simulink model "ICE_sim"  (R2026a)
settings: Solver=VariableStepAuto
PreLoadFcn:
  | % 模型加载前优先将当前目录与父目录加入 MATLAB 路径
  | modelPath = get_param(bdroot, 'FileName');
  | if ~isempty(modelPath)
  |     modelDir = fileparts(modelPath);
  |     addpath(modelDir);
  |     addpath(fullfile(modelDir, '..'));
  | end
InitFcn:
  | % 仅保留参数加载
  | common_params_init;
  | ice_params_init;
values from neighbouring files (symbols this model uses):
  BSFC_kg_per_kWh = Simulink.Parameter(0.24)    [ice_params_init.m]
  Critical_Overheat_Threshold_C = Simulink.Parameter(135)    [ice_params_init.m]
  Driveline_Efficiency = Simulink.Parameter(0.95)    [ice_params_init.m]
  Engine_HeatLossCoeff = Simulink.Parameter(0.1)    [ice_params_init.m]
  Engine_Temp_Init_C = Simulink.Parameter(40)    [ice_params_init.m]
  Engine_ThermalMass_JperC = Simulink.Parameter(50000)    [ice_params_init.m]
  Final_Drive_Ratio = Simulink.Parameter(3.5)    [ice_params_init.m]
  Fuel_Cut_RPM_Threshold = Simulink.Parameter(5000)    [ice_params_init.m]
  Fuel_Cut_Throttle_Threshold = Simulink.Parameter(5)    [ice_params_init.m]
  Fuel_Flow_Max_kg_s = Simulink.Parameter(0.028)    [ice_params_init.m]
  Fuel_LHV_J_per_kg = Simulink.Parameter(44e6)    [ice_params_init.m]
  Gear_Ratios = Simulink.Parameter([2.9 2.4 2.0 1.7 1.45 1.25 1.1 1.0])    [ice_params_init.m]
  Heat_Fraction_Coeff = Simulink.Parameter(0.3)    [ice_params_init.m]
  ICE_Max_Power_W = Simulink.Parameter(400000)    [ice_params_init.m]
  ICE_Max_Torque_Nm = Simulink.Parameter(320)    [ice_params_init.m]
  Idle_RPM_Threshold = Simulink.Parameter(4000)    [ice_params_init.m]
  Max_Safe_Boost_kPa = Simulink.Parameter(250)    [ice_params_init.m]
  Overheat_Threshold_C = Simulink.Parameter(105)    [ice_params_init.m]
  Race_Fuel_Limit_kg = Simulink.Parameter(110)    [ice_params_init.m]
  Shift_Down_RPM = Simulink.Parameter(9000)    [ice_params_init.m]
  Shift_Up_RPM = Simulink.Parameter(14500)    [ice_params_init.m]
  Throttle_Actuator_TimeConstant_s = Simulink.Parameter(0.05)    [ice_params_init.m]
  Turbo_FeedForward_Gain_Kff = Simulink.Parameter(1.0)    [ice_params_init.m]
  Turbo_FeedForward_Gain_Kff_Boosted = Simulink.Parameter(1.2)    [ice_params_init.m]
  Turbo_PID_Ki = Simulink.Parameter(0.1)    [ice_params_init.m]
  Turbo_PID_Kp = Simulink.Parameter(0.5)    [ice_params_init.m]
undefined symbols (not defined in the file or in its folder): Ambient_Temp_C, Wheel_Radius_m
libraries: simulink x1, sl_discontinuities x1, slpidlib x1
settings Model: Creator=nixiaofeng  LastModifiedBy=nixiaofeng

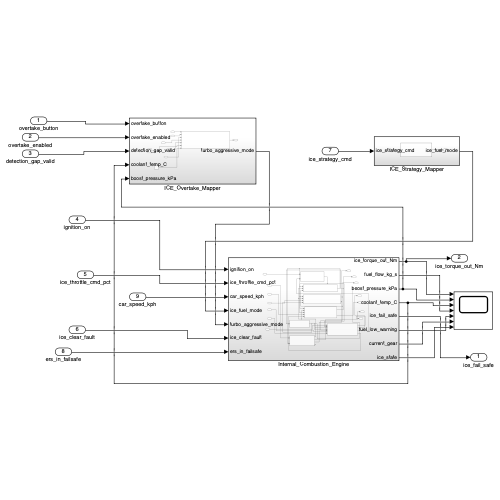
[thumbnail: Simulink's stored preview of the top-level diagram]
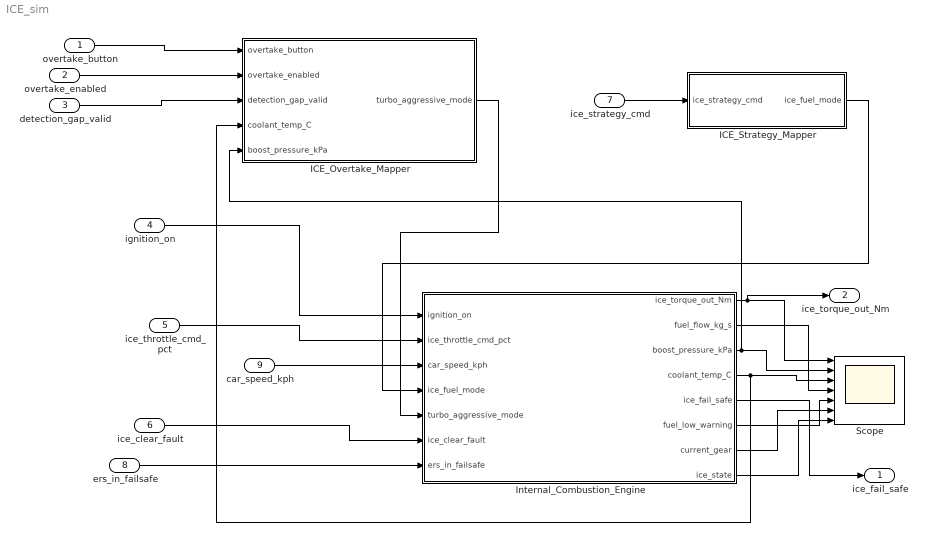
== system ICE_sim ==
  overtake_button : Inport
  overtake_enabled : Inport  Port=2
  detection_gap_valid : Inport  Port=3
  ignition_on : Inport  Port=4
  ice_throttle_cmd_pct : Inport  Port=5
  ice_clear_fault : Inport  Port=6
  ice_strategy_cmd : Inport  Port=7
  ers_in_failsafe : Inport  Port=8
  car_speed_kph : Inport  Port=9
  ICE_Overtake_Mapper : Subsystem
  ICE_Strategy_Mapper : Subsystem
  Internal_Combustion_Engine : Subsystem
  Scope : Scope  NumInputPorts=7
      settings: ActiveDisplayYMinimum=-5.6320436426453142  ActiveDisplayYMaximum=16.057146643170498
  ice_fail_safe : Outport
  ice_torque_out_Nm : Outport  Port=2
  wires:
  Internal_Combustion_Engine/1(ice_torque_out_Nm) -> ice_torque_out_Nm/1, Scope/1
  Internal_Combustion_Engine/3(boost_pressure_kPa) -> Scope/2, ICE_Overtake_Mapper/5(boost_pressure_kPa)
  Internal_Combustion_Engine/4(coolant_temp_C) -> ICE_Overtake_Mapper/4(coolant_temp_C), Scope/3
  Internal_Combustion_Engine/6(fuel_low_warning) -> Scope/5
  Internal_Combustion_Engine/2(fuel_flow_kg_s) -> Scope/4
  Internal_Combustion_Engine/7(current_gear) -> Scope/6
  Internal_Combustion_Engine/8(ice_state) -> Scope/7
  ICE_Strategy_Mapper/1(ice_fuel_mode) -> Internal_Combustion_Engine/4(ice_fuel_mode)
  ICE_Overtake_Mapper/1(turbo_aggressive_mode) -> Internal_Combustion_Engine/5(turbo_aggressive_mode)
  Internal_Combustion_Engine/5(ice_fail_safe) -> ice_fail_safe/1
  overtake_button/1 -> ICE_Overtake_Mapper/1(overtake_button)
  overtake_enabled/1 -> ICE_Overtake_Mapper/2(overtake_enabled)
  detection_gap_valid/1 -> ICE_Overtake_Mapper/3(detection_gap_valid)
  ignition_on/1 -> Internal_Combustion_Engine/1(ignition_on)
  ice_throttle_cmd_pct/1 -> Internal_Combustion_Engine/2(ice_throttle_cmd_pct)
  ice_clear_fault/1 -> Internal_Combustion_Engine/6(ice_clear_fault)
  ice_strategy_cmd/1 -> ICE_Strategy_Mapper/1(ice_strategy_cmd)
  ers_in_failsafe/1 -> Internal_Combustion_Engine/7(ers_in_failsafe)
  car_speed_kph/1 -> Internal_Combustion_Engine/3(car_speed_kph)

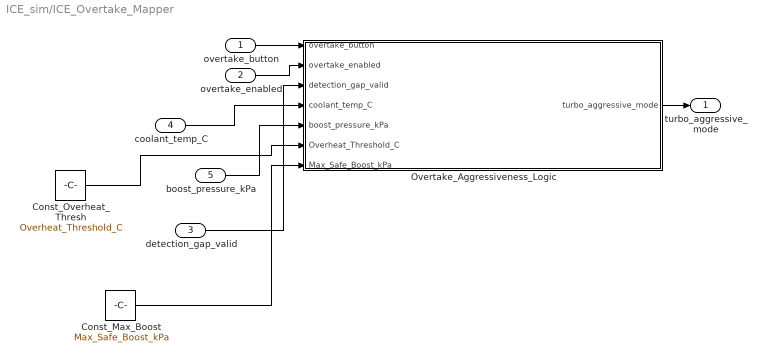
== system ICE_sim/ICE_Overtake_Mapper ==
  overtake_button : Inport
  overtake_enabled : Inport  Port=2
  detection_gap_valid : Inport  Port=3
  coolant_temp_C : Inport  Port=4
  boost_pressure_kPa : Inport  Port=5
  Const_Max_Boost : Constant  Value=Max_Safe_Boost_kPa
  Const_Overheat_Thresh : Constant  Value=Overheat_Threshold_C
  Overtake_Aggressiveness_Logic : MATLAB Function  TreatAsAtomicUnit=on
  turbo_aggressive_mode : Outport
  wires:
  overtake_button/1 -> Overtake_Aggressiveness_Logic/1(overtake_button)
  overtake_enabled/1 -> Overtake_Aggressiveness_Logic/2(overtake_enabled)
  detection_gap_valid/1 -> Overtake_Aggressiveness_Logic/3(detection_gap_valid)
  coolant_temp_C/1 -> Overtake_Aggressiveness_Logic/4(coolant_temp_C)
  boost_pressure_kPa/1 -> Overtake_Aggressiveness_Logic/5(boost_pressure_kPa)
  Const_Overheat_Thresh/1 -> Overtake_Aggressiveness_Logic/6(Overheat_Threshold_C)
  Const_Max_Boost/1 -> Overtake_Aggressiveness_Logic/7(Max_Safe_Boost_kPa)
  Overtake_Aggressiveness_Logic/1(turbo_aggressive_mode) -> turbo_aggressive_mode/1

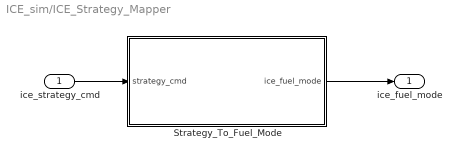
== system ICE_sim/ICE_Strategy_Mapper ==
  ice_strategy_cmd : Inport
  Strategy_To_Fuel_Mode : MATLAB Function  TreatAsAtomicUnit=on
  ice_fuel_mode : Outport
  wires:
  ice_strategy_cmd/1 -> Strategy_To_Fuel_Mode/1(strategy_cmd)
  Strategy_To_Fuel_Mode/1(ice_fuel_mode) -> ice_fuel_mode/1

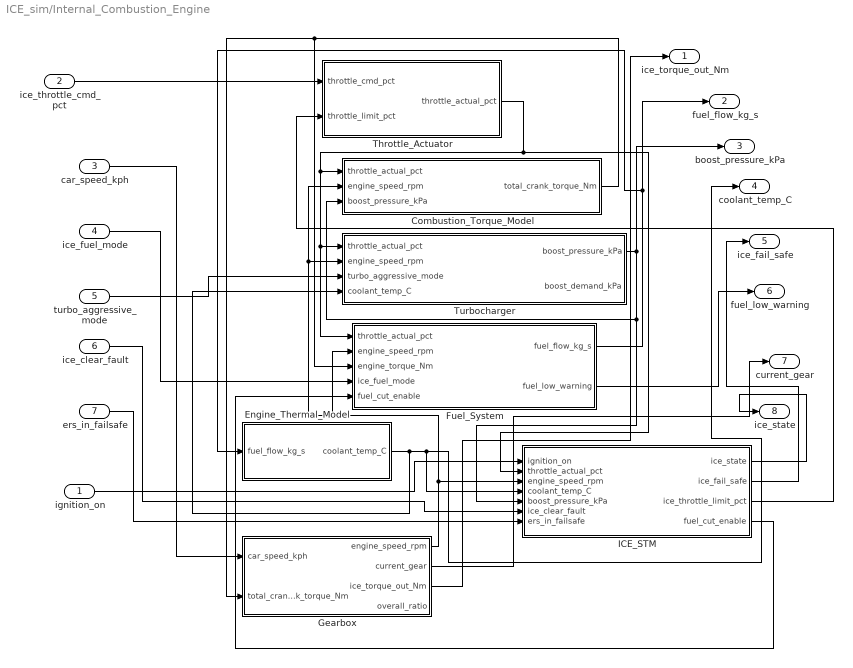
== system ICE_sim/Internal_Combustion_Engine ==
  ignition_on : Inport  OutDataTypeStr=boolean
  ice_throttle_cmd_pct : Inport  Port=2
  car_speed_kph : Inport  Port=3
  ice_fuel_mode : Inport  Port=4
  turbo_aggressive_mode : Inport  Port=5  OutDataTypeStr=boolean
  ice_clear_fault : Inport  Port=6  OutDataTypeStr=boolean
  ers_in_failsafe : Inport  Port=7  OutDataTypeStr=boolean
  Combustion_Torque_Model : Subsystem
  Engine_Thermal_Model : Subsystem
  Fuel_System : Subsystem
  Gearbox : Subsystem
  ICE_STM : Subsystem
  Throttle_Actuator : Subsystem
  Turbocharger : Subsystem
  ice_torque_out_Nm : Outport
  fuel_flow_kg_s : Outport  Port=2
  boost_pressure_kPa : Outport  Port=3
  coolant_temp_C : Outport  Port=4
  ice_fail_safe : Outport  Port=5
  fuel_low_warning : Outport  Port=6
  current_gear : Outport  Port=7
  ice_state : Outport  Port=8
  wires:
  ice_throttle_cmd_pct/1 -> Throttle_Actuator/1(throttle_cmd_pct)
  Throttle_Actuator/1(throttle_actual_pct) -> ICE_STM/2(throttle_actual_pct), Fuel_System/1(throttle_actual_pct), Turbocharger/1(throttle_actual_pct), Combustion_Torque_Model/1(throttle_actual_pct)
  ICE_STM/3(ice_throttle_limit_pct) -> Throttle_Actuator/2(throttle_limit_pct)
  Gearbox/1(engine_speed_rpm) -> ICE_STM/3(engine_speed_rpm), Fuel_System/2(engine_speed_rpm), Turbocharger/2(engine_speed_rpm), Combustion_Torque_Model/2(engine_speed_rpm)
  ignition_on/1 -> ICE_STM/1(ignition_on)
  Turbocharger/1(boost_pressure_kPa) -> ICE_STM/5(boost_pressure_kPa), Combustion_Torque_Model/3(boost_pressure_kPa), boost_pressure_kPa/1
  turbo_aggressive_mode/1 -> Turbocharger/3(turbo_aggressive_mode)
  Combustion_Torque_Model/1(total_crank_torque_Nm) -> Fuel_System/3(engine_torque_Nm), Gearbox/2(total_crank_torque_Nm)
  car_speed_kph/1 -> Gearbox/1(car_speed_kph)
  Gearbox/3(ice_torque_out_Nm) -> ice_torque_out_Nm/1
  Gearbox/2(current_gear) -> current_gear/1
  ice_fuel_mode/1 -> Fuel_System/4(ice_fuel_mode)
  ICE_STM/4(fuel_cut_enable) -> Fuel_System/5(fuel_cut_enable)
  Fuel_System/1(fuel_flow_kg_s) -> Engine_Thermal_Model/1(fuel_flow_kg_s), fuel_flow_kg_s/1
  Fuel_System/2(fuel_low_warning) -> fuel_low_warning/1
  Engine_Thermal_Model/1(coolant_temp_C) -> Turbocharger/4(coolant_temp_C), ICE_STM/4(coolant_temp_C), coolant_temp_C/1
  ice_clear_fault/1 -> ICE_STM/6(ice_clear_fault)
  ers_in_failsafe/1 -> ICE_STM/7(ers_in_failsafe)
  ICE_STM/1(ice_state) -> ice_state/1
  ICE_STM/2(ice_fail_safe) -> ice_fail_safe/1

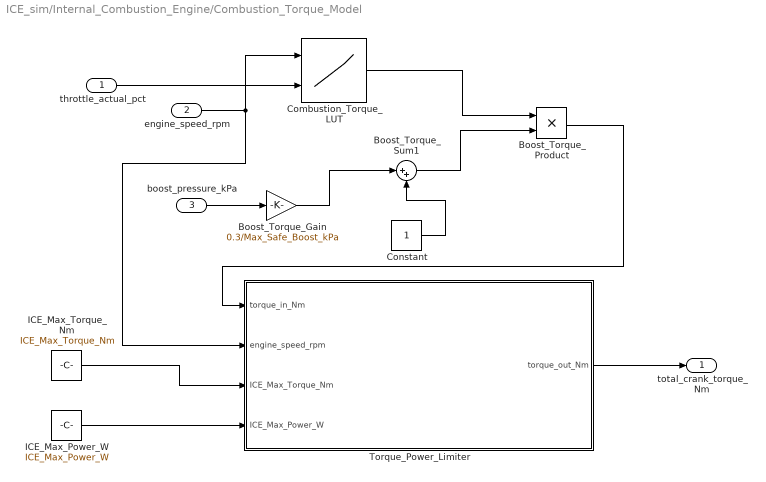
== system ICE_sim/Internal_Combustion_Engine/Combustion_Torque_Model ==
  throttle_actual_pct : Inport  Unit=%
  engine_speed_rpm : Inport  Port=2  Unit=rpm
  boost_pressure_kPa : Inport  Port=3  Unit=kPa
  Boost_Torque_Gain : Gain  Gain=0.3/Max_Safe_Boost_kPa
  Boost_Torque_Product : Product
  Boost_Torque_Sum1 : Sum  Inputs=|++
  Combustion_Torque_LUT : Lookup_n-D  BreakpointsForDimension1=[4000 6000 8000 10000 12000 14000 15000]  BreakpointsForDimension2=[0 20 40 60 80 100]  Table=|  InternalRulePriority=Speed  RndMeth=Simplest
      | [0 50 100 150 200 250;
      |  0 80 160 240 320 400;
      |  0 100 200 300 400 500;
      |  0 110 220 330 440 550;
      |  0 105 210 315 420 525;
      |  0 90 180 270 360 450;
      |  0 70 140 210 280 350]
      settings: InputPortMap=u0,u1
  Constant : Constant
  ICE_Max_Power_W : Constant  Value=ICE_Max_Power_W
  ICE_Max_Torque_Nm : Constant  Value=ICE_Max_Torque_Nm
  Torque_Power_Limiter : MATLAB Function  TreatAsAtomicUnit=on
  total_crank_torque_Nm : Outport  Unit=N*m
  wires:
  Constant/1 -> Boost_Torque_Sum1/2
  engine_speed_rpm/1 -> Torque_Power_Limiter/2(engine_speed_rpm), Combustion_Torque_LUT/1
  Combustion_Torque_LUT/1 -> Boost_Torque_Product/1
  boost_pressure_kPa/1 -> Boost_Torque_Gain/1
  Boost_Torque_Gain/1 -> Boost_Torque_Sum1/1
  Boost_Torque_Sum1/1 -> Boost_Torque_Product/2
  Torque_Power_Limiter/1(torque_out_Nm) -> total_crank_torque_Nm/1
  Boost_Torque_Product/1 -> Torque_Power_Limiter/1(torque_in_Nm)
  throttle_actual_pct/1 -> Combustion_Torque_LUT/2
  ICE_Max_Torque_Nm/1 -> Torque_Power_Limiter/3(ICE_Max_Torque_Nm)
  ICE_Max_Power_W/1 -> Torque_Power_Limiter/4(ICE_Max_Power_W)

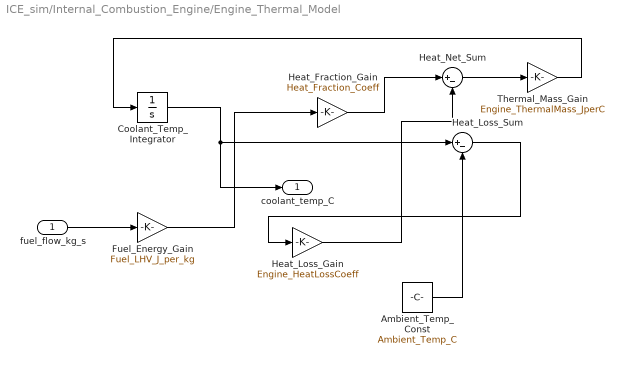
== system ICE_sim/Internal_Combustion_Engine/Engine_Thermal_Model ==
  fuel_flow_kg_s : Inport
  Ambient_Temp_Const : Constant  Value=Ambient_Temp_C
  Coolant_Temp_Integrator : Integrator  InitialCondition=Engine_Temp_Init_C
  Fuel_Energy_Gain : Gain  Gain=Fuel_LHV_J_per_kg
  Heat_Fraction_Gain : Gain  Gain=Heat_Fraction_Coeff
  Heat_Loss_Gain : Gain  Gain=Engine_HeatLossCoeff
  Heat_Loss_Sum : Sum  Inputs=|+-
  Heat_Net_Sum : Sum  Inputs=|+-
  Thermal_Mass_Gain : Gain  Gain=Engine_ThermalMass_JperC
  coolant_temp_C : Outport
  wires:
  fuel_flow_kg_s/1 -> Fuel_Energy_Gain/1
  Fuel_Energy_Gain/1 -> Heat_Fraction_Gain/1
  Heat_Fraction_Gain/1 -> Heat_Net_Sum/1
  Coolant_Temp_Integrator/1 -> coolant_temp_C/1, Heat_Loss_Sum/1
  Ambient_Temp_Const/1 -> Heat_Loss_Sum/2
  Heat_Loss_Sum/1 -> Heat_Loss_Gain/1
  Heat_Loss_Gain/1 -> Heat_Net_Sum/2
  Heat_Net_Sum/1 -> Thermal_Mass_Gain/1
  Thermal_Mass_Gain/1 -> Coolant_Temp_Integrator/1

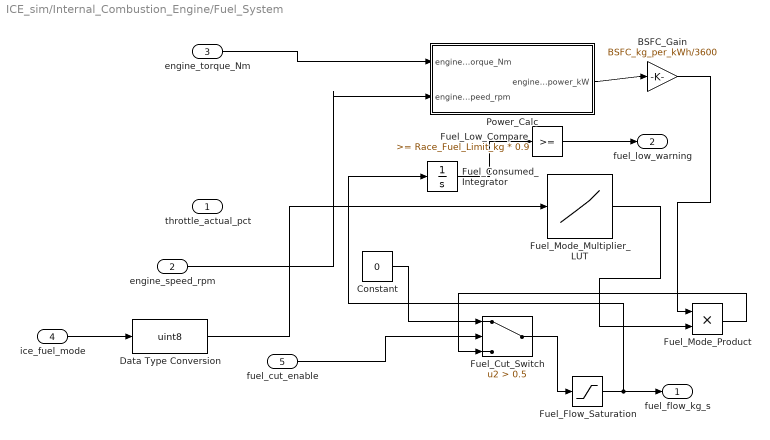
== system ICE_sim/Internal_Combustion_Engine/Fuel_System ==
  throttle_actual_pct : Inport
  engine_speed_rpm : Inport  Port=2
  engine_torque_Nm : Inport  Port=3
  ice_fuel_mode : Inport  Port=4
  fuel_cut_enable : Inport  Port=5
  BSFC_Gain : Gain  Gain=BSFC_kg_per_kWh/3600
  Constant : Constant  Value=0
  Data Type Conversion : DataTypeConversion  OutDataTypeStr=uint8  SaturateOnIntegerOverflow=off  RndMeth=Floor
  Fuel_Consumed_Integrator : Integrator
  Fuel_Cut_Switch : Switch  Criteria=u2 > Threshold  Threshold=0.5  SaturateOnIntegerOverflow=off  InputSameDT=off
  Fuel_Flow_Saturation : Saturate  UpperLimit=Fuel_Flow_Max_kg_s  LowerLimit=0
  Fuel_Low_Compare : simulink/Logic and Bit Operations/Compare To Constant  relop=>=  const=Race_Fuel_Limit_kg * 0.9  OutDataTypeStr=boolean
  Fuel_Mode_Multiplier_LUT : Lookup_n-D  NumberOfTableDimensions=1  BreakpointsForDimension1=[0 1 2]  BreakpointsForDimension1DataTypeStr=Inherit: Inherit from 'Breakpoint data'  Table=[1.0 0.75 0.55]  ExtrapMethod=Clip  InternalRulePriority=Speed  OutDataTypeStr=double  RndMeth=Simplest
  Fuel_Mode_Product : Product
  Power_Calc : Subsystem
  fuel_flow_kg_s : Outport
  fuel_low_warning : Outport  Port=2
  wires:
  engine_torque_Nm/1 -> Power_Calc/1(engine_torque_Nm)
  engine_speed_rpm/1 -> Power_Calc/2(engine_speed_rpm)
  Power_Calc/1(engine_power_kW) -> BSFC_Gain/1
  BSFC_Gain/1 -> Fuel_Mode_Product/1
  Fuel_Mode_Multiplier_LUT/1 -> Fuel_Mode_Product/2
  Constant/1 -> Fuel_Cut_Switch/1
  fuel_cut_enable/1 -> Fuel_Cut_Switch/2
  Fuel_Mode_Product/1 -> Fuel_Cut_Switch/3
  Fuel_Cut_Switch/1 -> Fuel_Flow_Saturation/1
  Fuel_Flow_Saturation/1 -> Fuel_Consumed_Integrator/1, fuel_flow_kg_s/1
  Fuel_Consumed_Integrator/1 -> Fuel_Low_Compare/1
  Fuel_Low_Compare/1 -> fuel_low_warning/1
  ice_fuel_mode/1 -> Data Type Conversion/1
  Data Type Conversion/1 -> Fuel_Mode_Multiplier_LUT/1

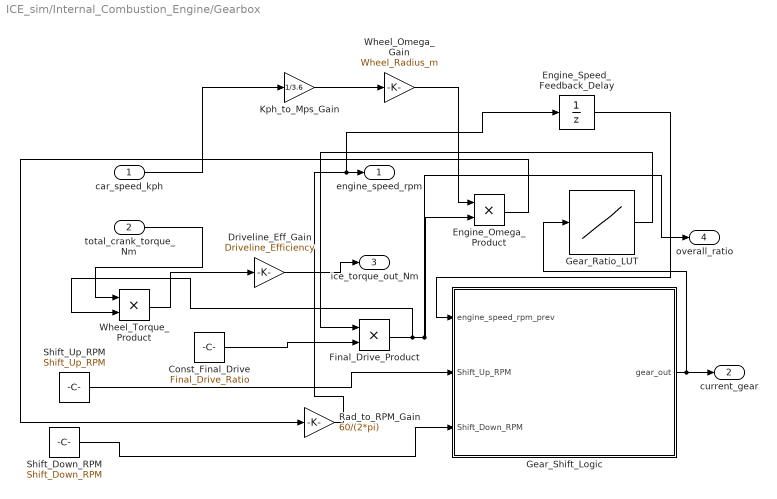
== system ICE_sim/Internal_Combustion_Engine/Gearbox ==
  car_speed_kph : Inport
  total_crank_torque_Nm : Inport  Port=2
  Const_Final_Drive : Constant  Value=Final_Drive_Ratio
  Driveline_Eff_Gain : Gain  Gain=Driveline_Efficiency
  Engine_Omega_Product : Product
  Engine_Speed_Feedback_Delay : UnitDelay  InitialCondition=Idle_RPM_Threshold  SampleTime=-1
  Final_Drive_Product : Product
  Gear_Ratio_LUT : Lookup_n-D  NumberOfTableDimensions=1  BreakpointsForDimension1=[1 2 3 4 5 6 7 8]  Table=Gear_Ratios  TableDataTypeStr=Inherit: Inherit from 'Table data'  ExtrapMethod=Clip  InternalRulePriority=Speed  OutDataTypeStr=double  RndMeth=Simplest
  Gear_Shift_Logic : MATLAB Function  TreatAsAtomicUnit=on
  Kph_to_Mps_Gain : Gain  Gain=1/3.6
  Rad_to_RPM_Gain : Gain  Gain=60/(2*pi)
  Shift_Down_RPM : Constant  Value=Shift_Down_RPM
  Shift_Up_RPM : Constant  Value=Shift_Up_RPM
  Wheel_Omega_Gain : Gain  Gain=Wheel_Radius_m
  Wheel_Torque_Product : Product
  engine_speed_rpm : Outport
  current_gear : Outport  Port=2
  ice_torque_out_Nm : Outport  Port=3
  overall_ratio : Outport  Port=4
  wires:
  Shift_Up_RPM/1 -> Gear_Shift_Logic/2(Shift_Up_RPM)
  Shift_Down_RPM/1 -> Gear_Shift_Logic/3(Shift_Down_RPM)
  Engine_Speed_Feedback_Delay/1 -> Gear_Shift_Logic/1(engine_speed_rpm_prev)
  Gear_Shift_Logic/1(gear_out) -> Gear_Ratio_LUT/1, current_gear/1
  Gear_Ratio_LUT/1 -> Final_Drive_Product/1
  Const_Final_Drive/1 -> Final_Drive_Product/2
  car_speed_kph/1 -> Kph_to_Mps_Gain/1
  Kph_to_Mps_Gain/1 -> Wheel_Omega_Gain/1
  Wheel_Omega_Gain/1 -> Engine_Omega_Product/1
  Final_Drive_Product/1 -> Wheel_Torque_Product/2, overall_ratio/1, Engine_Omega_Product/2
  Engine_Omega_Product/1 -> Rad_to_RPM_Gain/1
  Rad_to_RPM_Gain/1 -> Engine_Speed_Feedback_Delay/1, engine_speed_rpm/1
  total_crank_torque_Nm/1 -> Wheel_Torque_Product/1
  Wheel_Torque_Product/1 -> Driveline_Eff_Gain/1
  Driveline_Eff_Gain/1 -> ice_torque_out_Nm/1

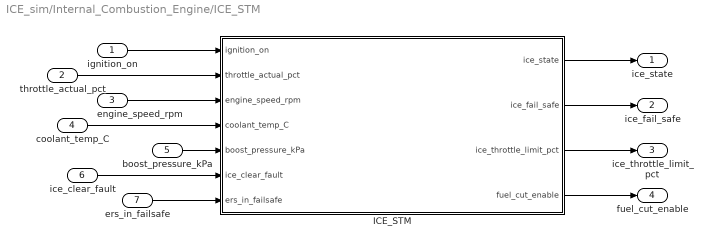
== system ICE_sim/Internal_Combustion_Engine/ICE_STM ==
  ignition_on : Inport
  throttle_actual_pct : Inport  Port=2
  engine_speed_rpm : Inport  Port=3
  coolant_temp_C : Inport  Port=4
  boost_pressure_kPa : Inport  Port=5
  ice_clear_fault : Inport  Port=6
  ers_in_failsafe : Inport  Port=7
  ICE_STM : Stateflow chart  TreatAsAtomicUnit=on
  ice_state : Outport
  ice_fail_safe : Outport  Port=2
  ice_throttle_limit_pct : Outport  Port=3
  fuel_cut_enable : Outport  Port=4
  wires:
  ignition_on/1 -> ICE_STM/1(ignition_on)
  throttle_actual_pct/1 -> ICE_STM/2(throttle_actual_pct)
  engine_speed_rpm/1 -> ICE_STM/3(engine_speed_rpm)
  coolant_temp_C/1 -> ICE_STM/4(coolant_temp_C)
  boost_pressure_kPa/1 -> ICE_STM/5(boost_pressure_kPa)
  ice_clear_fault/1 -> ICE_STM/6(ice_clear_fault)
  ers_in_failsafe/1 -> ICE_STM/7(ers_in_failsafe)
  ICE_STM/1(ice_state) -> ice_state/1
  ICE_STM/2(ice_fail_safe) -> ice_fail_safe/1
  ICE_STM/3(ice_throttle_limit_pct) -> ice_throttle_limit_pct/1
  ICE_STM/4(fuel_cut_enable) -> fuel_cut_enable/1

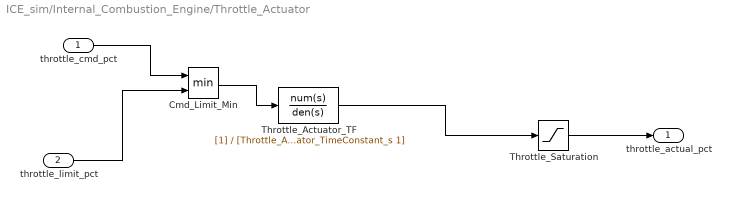
== system ICE_sim/Internal_Combustion_Engine/Throttle_Actuator ==
  throttle_cmd_pct : Inport  Unit=%
  throttle_limit_pct : Inport  Port=2  Unit=%
  Cmd_Limit_Min : MinMax  Inputs=2
  Throttle_Actuator_TF : TransferFcn  Denominator=[Throttle_Actuator_TimeConstant_s 1]
  Throttle_Saturation : Saturate  UpperLimit=100  LowerLimit=0
  throttle_actual_pct : Outport  Unit=%
  wires:
  throttle_cmd_pct/1 -> Cmd_Limit_Min/1
  throttle_limit_pct/1 -> Cmd_Limit_Min/2
  Cmd_Limit_Min/1 -> Throttle_Actuator_TF/1
  Throttle_Actuator_TF/1 -> Throttle_Saturation/1
  Throttle_Saturation/1 -> throttle_actual_pct/1

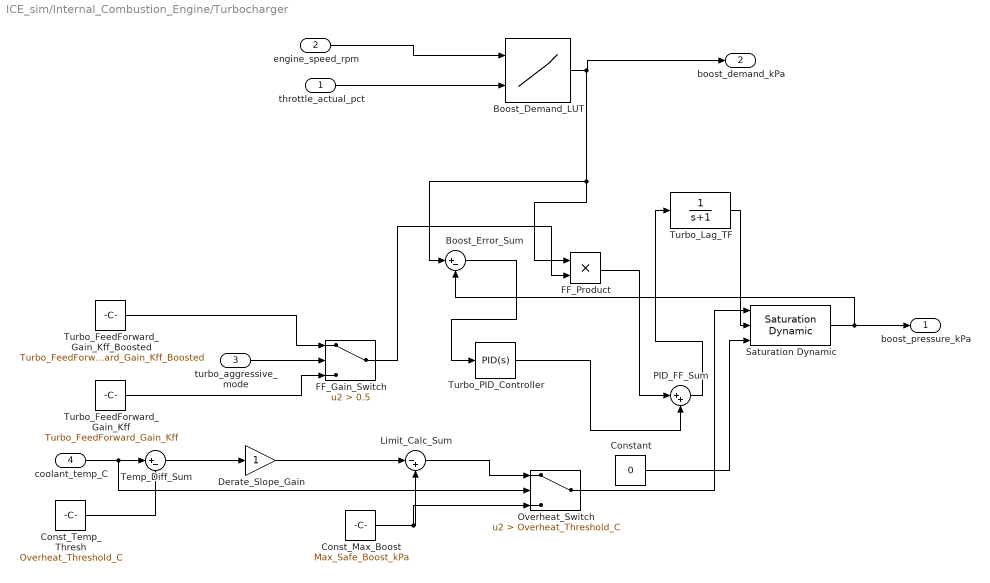
== system ICE_sim/Internal_Combustion_Engine/Turbocharger ==
  throttle_actual_pct : Inport
  engine_speed_rpm : Inport  Port=2
  turbo_aggressive_mode : Inport  Port=3
  coolant_temp_C : Inport  Port=4
  Boost_Demand_LUT : Lookup_n-D  BreakpointsForDimension1=[4000 6000 8000 10000 12000 14000 15000]  BreakpointsForDimension2=[0 20 40 60 80 100]  Table=|  InternalRulePriority=Speed  RndMeth=Simplest
      | [ 0  10   30   60   90  120;
      |   0  20   50  100  140  180;
      |   0  30   70  130  180  220;
      |   0  40   80  150  200  250;
      |   0  40   80  150  200  250;
      |   0  35   70  130  180  220;
      |   0  20   50  100  140  180 ]
      settings: InputPortMap=u0,u1
  Boost_Error_Sum : Sum  Inputs=|+-
  Const_Max_Boost : Constant  Value=Max_Safe_Boost_kPa
  Const_Temp_Thresh : Constant  Value=Overheat_Threshold_C
  Constant : Constant  Value=0
  Derate_Slope_Gain : Gain
  FF_Gain_Switch : Switch  Criteria=u2 > Threshold  Threshold=0.5  SaturateOnIntegerOverflow=off  InputSameDT=off
  FF_Product : Product
  Limit_Calc_Sum : Sum  Inputs=|-+
  Overheat_Switch : Switch  Criteria=u2 > Threshold  Threshold=Overheat_Threshold_C  SaturateOnIntegerOverflow=off  InputSameDT=off
  PID_FF_Sum : Sum  Inputs=|++
  Saturation Dynamic : sl_discontinuities/Saturation Dynamic  OutMin=[]  OutMax=[]  OutDataTypeStr=Inherit: Same as second input  OutDataType=fixdt(1, 16)  OutScaling=2^-10  DoSatur=off
      settings: LibrarySourceBlock=|
      | simulink/Discontinuities/Saturation
      | Dynamic
  Temp_Diff_Sum : Sum  Inputs=|+-
  Turbo_FeedForward_Gain_Kff : Constant  Value=Turbo_FeedForward_Gain_Kff
  Turbo_FeedForward_Gain_Kff_Boosted : Constant  Value=Turbo_FeedForward_Gain_Kff_Boosted
  Turbo_Lag_TF : TransferFcn  Denominator=[1 1]
  Turbo_PID_Controller : slpidlib/PID Controller  Controller=PID  Form=Parallel  TimeDomain=Continuous-time  UseExternalTs=off  SampleTime=-1  IntegratorMethod=Forward Euler  FilterMethod=Forward Euler  ControllerParametersSource=internal  P=Turbo_PID_Kp  I=Turbo_PID_Ki  UseKiTs=off  D=0  UseExternalDerivativeSource=off  N=100  UseFilter=on  TunerSelectOption=Transfer Function Based (PID Tuner App)  InitialConditionSource=internal  InitialConditionForIntegrator=0  InitialConditionForFilter=0  DifferentiatorICPrevScaledInput=0  ExternalReset=none  TrackingMode=off  Kt=1  LimitOutput=off  SatLimitsSource=internal  UpperSaturationLimit=inf  LowerSaturationLimit=-inf  LinearizeAsGain=on  AntiWindupMode=none  Kb=1  LimitIntegrator=off  UpperIntegratorSaturationLimit=inf  LowerIntegratorSaturationLimit=-inf  POutMin=[]  POutMax=[]  IOutMin=[]  IOutMax=[]  DOutMin=[]  DOutMax=[]  NOutMin=[]  NOutMax=[]  SumOutMin=[]  SumOutMax=[]  SaturationOutMin=[]  SaturationOutMax=[]  PParamMin=[]  PParamMax=[]  IParamMin=[]  IParamMax=[]  DParamMin=[]  DParamMax=[]  NParamMin=[]  NParamMax=[]  KbParamMin=[]  KbParamMax=[]  KtParamMin=[]  KtParamMax=[]  KbOutMin=[]  KbOutMax=[]  KtOutMin=[]  KtOutMax=[]  IntegratorOutMin=[]  IntegratorOutMax=[]  FilterOutMin=[]  FilterOutMax=[]  SumI1OutMin=[]  SumI1OutMax=[]  SumI2OutMin=[]  SumI2OutMax=[]  SumI3OutMin=[]  SumI3OutMax=[]  SumI4OutMin=[]  SumI4OutMax=[]  SumDOutMin=[]  SumDOutMax=[]  DifferentiatorOutMin=[]  DifferentiatorOutMax=[]  FilterDiffOutCoefMin=[]  FilterDiffOutCoefMax=[]  ReciprocalOutMin=[]  ReciprocalOutMax=[]  SumDenOutMin=[]  SumDenOutMax=[]  SumNumOutMin=[]  SumNumOutMax=[]  DivideOutMin=[]  DivideOutMax=[]  UdiffTsProdOutMin=[]  UdiffTsProdOutMax=[]  NTsProdOutMin=[]  NTsProdOutMax=[]  UintegralTsProdOutMin=[]  UintegralTsProdOutMax=[]  UngainTsProdOutMin=[]  UngainTsProdOutMax=[]  ClampingZeroOutDataTypeStr=Inherit: Inherit via back propagation  ClampingZeroOutMin=[]  ClampingZeroOutMax=[]  FilterDenConstantOutDataTypeStr=Inherit: Inherit via back propagation  FilterDenConstantOutMin=[]  FilterDenConstantOutMax=[]  PCopyOutDataTypeStr=Inherit: Inherit via back propagation  PCopyOutMin=[]  PCopyOutMax=[]  NCopyOutDataTypeStr=Inherit: Inherit via back propagation  NCopyOutMin=[]  NCopyOutMax=[]  IntegratorContinuousStateAttributes=''  IntegratorStateMustResolveToSignalObject=off  IntegratorRTWStateStorageClass=Auto  FilterContinuousStateAttributes=''  FilterStateMustResolveToSignalObject=off  FilterRTWStateStorageClass=Auto  ParallelPVariant=InternalParameters  IdealPVariant=Disabled  IVariant=InternalParameters  DVariant=InternalParameters  IntegratorVariant=Continuous  SatVariant=Disabled  AWVariant=Passthrough  PCopyVariant=Disabled  TRVariant=Disabled  FdbkBlocksVariant=Forward  IdealPFdbkVariant=Disabled  SatFdbkVariant=Disabled  DerivativeFilterVariant=ContFilter  NVariant=InternalParameters  NCopyVariant=Disabled  FilterICVariant=InternalICsFilter  IntegratorICVariant=InternalICs  ExternalResetVariant=Disabled  TRSumVariant=Passthrough  SumFdbkVariant=Disabled  SumVariant=Sum_PID  TsampFilterVariant=InternalTs  TsampNgainVariant=Passthrough  TsampIntegralVariant=Disabled_SignalSpec  ExternalSaturationOutDataTypeStr=Inherit: Same as second input  DerivativeSourceVariant=ErrorSignal  PreIntVariant=InternalPreInt
  boost_pressure_kPa : Outport
  boost_demand_kPa : Outport  Port=2
  wires:
  engine_speed_rpm/1 -> Boost_Demand_LUT/1
  throttle_actual_pct/1 -> Boost_Demand_LUT/2
  Boost_Demand_LUT/1 -> FF_Product/1, Boost_Error_Sum/1, boost_demand_kPa/1
  turbo_aggressive_mode/1 -> FF_Gain_Switch/2
  Turbo_FeedForward_Gain_Kff_Boosted/1 -> FF_Gain_Switch/1
  Turbo_FeedForward_Gain_Kff/1 -> FF_Gain_Switch/3
  Turbo_Lag_TF/1 -> Saturation Dynamic/2
  Saturation Dynamic/1 -> boost_pressure_kPa/1, Boost_Error_Sum/2
  Constant/1 -> Saturation Dynamic/3
  coolant_temp_C/1 -> Overheat_Switch/2, Temp_Diff_Sum/1
  Const_Temp_Thresh/1 -> Temp_Diff_Sum/2
  Temp_Diff_Sum/1 -> Derate_Slope_Gain/1
  Derate_Slope_Gain/1 -> Limit_Calc_Sum/1
  Const_Max_Boost/1 -> Overheat_Switch/3, Limit_Calc_Sum/2
  Limit_Calc_Sum/1 -> Overheat_Switch/1
  Overheat_Switch/1 -> Saturation Dynamic/1
  Boost_Error_Sum/1 -> Turbo_PID_Controller/1
  FF_Gain_Switch/1 -> FF_Product/2
  FF_Product/1 -> PID_FF_Sum/1
  Turbo_PID_Controller/1 -> PID_FF_Sum/2
  PID_FF_Sum/1 -> Turbo_Lag_TF/1

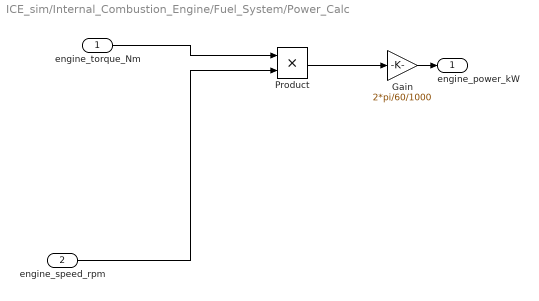
== system ICE_sim/Internal_Combustion_Engine/Fuel_System/Power_Calc ==
  engine_torque_Nm : Inport
  engine_speed_rpm : Inport  Port=2
  Gain : Gain  Gain=2*pi/60/1000
  Product : Product
  engine_power_kW : Outport
  wires:
  engine_torque_Nm/1 -> Product/1
  engine_speed_rpm/1 -> Product/2
  Gain/1 -> engine_power_kW/1
  Product/1 -> Gain/1

== matlab function ICE_sim/ICE_Strategy_Mapper/Strategy_To_Fuel_Mode ==
  data: strategy_cmd input; ice_fuel_mode output
function ice_fuel_mode = Strategy_To_Fuel_Mode(strategy_cmd)
    % 策略指令映射逻辑 (示例编码：0=Race, 1=Push, 2=Charge, 3=Save)
    switch double(strategy_cmd)
        case 0   % Race (标准正赛)
            ice_fuel_mode = ICE_Fuel_Mode.Normal;
        case 1   % Push (排位/超车激进模式)
            ice_fuel_mode = ICE_Fuel_Mode.Normal;
        case 2   % Charge (巡航充能/保油)
            ice_fuel_mode = ICE_Fuel_Mode.Fuel_Saving;
        case 3   % Lift & Coast (抬油门滑行)
            ice_fuel_mode = ICE_Fuel_Mode.Lift_and_Coast;
        otherwise
            ice_fuel_mode = ICE_Fuel_Mode.Normal;
    end
end

== matlab function ICE_sim/ICE_Overtake_Mapper/Overtake_Aggressiveness_Logic ==
  data: overtake_button input; turbo_aggressive_mode output; overtake_enabled input; detection_gap_valid input; coolant_temp_C input; boost_pressure_kPa input; Overheat_Threshold_C input; Max_Safe_Boost_kPa input
function turbo_aggressive_mode = Overtake_Aggressiveness_Logic( ...
        overtake_button, overtake_enabled, detection_gap_valid, ...
        coolant_temp_C, boost_pressure_kPa, ...
        Overheat_Threshold_C, Max_Safe_Boost_kPa)

    % 1. 检查热裕度和增压裕度 (留出 5% 安全余量)
    thermal_margin_ok = coolant_temp_C < Overheat_Threshold_C;
    boost_margin_ok   = boost_pressure_kPa < (Max_Safe_Boost_kPa * 0.95);

    % 2. 综合判断是否开启涡轮激进模式
    turbo_aggressive_mode = overtake_button && overtake_enabled && ...
                            detection_gap_valid && thermal_margin_ok && boost_margin_ok;
end

== matlab function ICE_sim/Internal_Combustion_Engine/Gearbox/Gear_Shift_Logic ==
  data: engine_speed_rpm_prev input; gear_out output; Shift_Up_RPM input; Shift_Down_RPM input
function gear_out = Gear_Shift_Logic(engine_speed_rpm_prev, Shift_Up_RPM, Shift_Down_RPM)
    % 升降档状态保持变量
    persistent gear
    if isempty(gear)
        gear = uint8(1); % 初始状态默认 1 档
    end
    
    % 基于上一步转速的滞后换挡逻辑
    if engine_speed_rpm_prev >= Shift_Up_RPM && gear < 8
        gear = gear + 1;
    elseif engine_speed_rpm_prev <= Shift_Down_RPM && gear > 1
        gear = gear - 1;
    end
    
    gear_out = gear;
end

== matlab function ICE_sim/Internal_Combustion_Engine/Combustion_Torque_Model/Torque_Power_Limiter ==
  data: torque_in_Nm input; torque_out_Nm output; engine_speed_rpm input; ICE_Max_Torque_Nm input; ICE_Max_Power_W input
function torque_out_Nm = Torque_Power_Limiter(torque_in_Nm, engine_speed_rpm, ICE_Max_Torque_Nm, ICE_Max_Power_W)
    torque_capped = min(torque_in_Nm, ICE_Max_Torque_Nm);
    omega_rad_s = engine_speed_rpm * 2*pi/60;
    if omega_rad_s > 1e-3
        power_W = torque_capped * omega_rad_s;
        if power_W > ICE_Max_Power_W
            torque_capped = ICE_Max_Power_W / omega_rad_s;
        end
    end
    torque_out_Nm = max(torque_capped, 0);
end

== stateflow chart ICE_sim/Internal_Combustion_Engine/ICE_STM/ICE_STM ==
  state Operation_Modes
    state Cranking
      entry:
      ice_state = ICE_State.Cranking;
      ice_fail_safe = false;
      ice_throttle_limit_pct = 30;
      fuel_cut_enable = false;
    state Active_Modes
      state Idle
        entry:
        ice_state = ICE_State.Idle;
        ice_fail_safe = false;
        ice_throttle_limit_pct = 100;
        fuel_cut_enable = false;
      state Running
        entry:
        ice_state = ICE_State.Running;
        ice_fail_safe = false;
        ice_throttle_limit_pct = 100;
        fuel_cut_enable = false;
      state Fuel_Cut
        entry:
        ice_state = ICE_State.Fuel_Cut;
        ice_fail_safe = false;
        ice_throttle_limit_pct = 100;
        fuel_cut_enable = true;
      Running -> Idle [order 1] : [throttle_actual_pct <= Fuel_Cut_Throttle_Threshold && engine_speed_rpm <= Idle_RPM_Threshold]
      Idle -> Running : [throttle_actual_pct > Fuel_Cut_Throttle_Threshold]
      Fuel_Cut -> Running : [throttle_actual_pct >= Fuel_Cut_Throttle_Threshold]
      Running -> Fuel_Cut [order 2] : [engine_speed_rpm > Fuel_Cut_RPM_Threshold && throttle_actual_pct < Fuel_Cut_Throttle_Threshold]
    Cranking -> Idle : [engine_speed_rpm > Idle_RPM_Threshold * 0.3]
  state Off_Standby
    entry:
    ice_state = ICE_State.Off_Standby;
    ice_fail_safe = false;
    ice_throttle_limit_pct = 0;
    fuel_cut_enable = false;
  state Limp_Home
    entry:
    ice_state = ICE_State.Limp_Home;
    ice_fail_safe = false;
    ice_throttle_limit_pct = 50;
    fuel_cut_enable = false;
  state Fail_Safe
    entry:
    ice_state = ICE_State.Fail_Safe;
    ice_fail_safe = true;
    ice_throttle_limit_pct = 0;
    fuel_cut_enable = true;
  (default) -> Off_Standby
  Off_Standby -> Cranking : [ignition_on == true]
  Fail_Safe -> Off_Standby : [ice_clear_fault == true]
  Limp_Home -> Running : [coolant_temp_C < (Overheat_Threshold_C - 5)]
  Active_Modes -> Limp_Home : [coolant_temp_C > Overheat_Threshold_C]
  Operation_Modes -> Fail_Safe : [coolant_temp_C > Critical_Overheat_Threshold_C || boost_pressure_kPa > Max_Safe_Boost_kPa || ers_in_failsafe == true]
  data: ignition_on input; throttle_actual_pct input; engine_speed_rpm input; coolant_temp_C input; boost_pressure_kPa input; ice_clear_fault input; ers_in_failsafe input; ice_state output; ice_fail_safe output; ice_throttle_limit_pct output; fuel_cut_enable output; Idle_RPM_Threshold parameter; Fuel_Cut_Throttle_Threshold parameter; Fuel_Cut_RPM_Threshold parameter; Overheat_Threshold_C parameter; Critical_Overheat_Threshold_C parameter; Max_Safe_Boost_kPa parameter
